simulink model "balanced_modelreduction_rlc"  (R2020b)
settings: Solver=FixedStepAuto  StartTime=0.0  StopTime=3  FixedStep=5e-7  RelTol=1e-3
values from neighbouring files (symbols this model uses):
  n = 20    [Model_1.mat]    (also in Model_11.mat = 100; Model_12.mat = 100; Model_13.mat = 100; Model_14.mat = 100)
undefined symbols (not defined in the file or in its folder): A, Ar, Arg, B, Br, Brg, C, Cr, Crg, K
settings Model: Creator=p282922  LastModifiedBy=S2940884
settings DataIOCC: ReturnWorkspaceOutputs=off
settings DebuggingCC: ArithmeticOperatorsInVariantConditions=warning
settings SFSimCC: SimUseLocalCustomCode=off  CustomCodeUndefinedFunction=UseInterfaceOnly
settings RTWCC: RTWUseLocalCustomCode=off

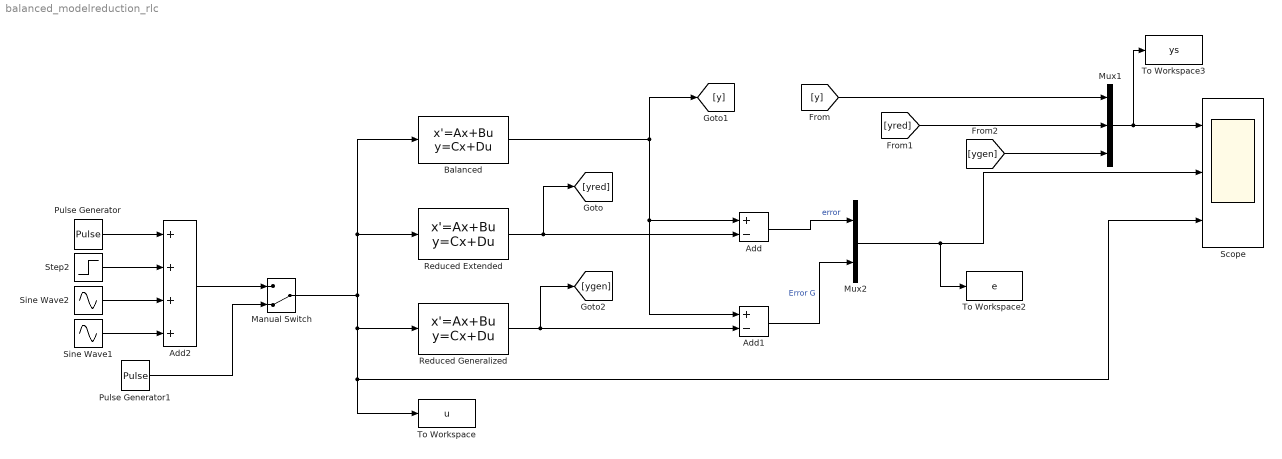
== system balanced_modelreduction_rlc ==
  Add : Sum  Inputs=+-
  Add1 : Sum  Inputs=+-
  Add2 : Sum  Inputs=++++
  Balanced : StateSpace  A=A  B=B  C=C  D=0  InitialCondition=zeros(2*n,1)
  Manual Switch : ManualSwitch  CurrentSetting=0
  Mux1 : Mux  Inputs=3
  Mux2 : Mux  Inputs=2
  Pulse Generator : DiscretePulseGenerator  PulseType=Time based  Amplitude=5  Period=1  PulseWidth=50
  Pulse Generator1 : DiscretePulseGenerator  PulseType=Time based  Amplitude=50  Period=1  PulseWidth=50
  Reduced Extended : StateSpace  A=Ar  B=Br  C=Cr  D=0  InitialCondition=zeros(K,1)
  Reduced Generalized : StateSpace  A=Arg  B=Brg  C=Crg  D=0  InitialCondition=zeros(K,1)
  Scope : Scope  NumInputPorts=3
  Sine Wave1 : Sin  Amplitude=12  Frequency=23  Phase=pi/2  SampleTime=0
  Sine Wave2 : Sin  Amplitude=9  Frequency=17  SampleTime=0
  Step2 : Step  Time=2  After=-30*0  SampleTime=0
  To Workspace : ToWorkspace  VariableName=u  SaveFormat=Structure With Time  SampleTime=-1
  To Workspace2 : ToWorkspace  VariableName=e  SaveFormat=Structure With Time  SampleTime=-1
  To Workspace3 : ToWorkspace  VariableName=ys  SaveFormat=Structure With Time  SampleTime=-1
  wires:
  Balanced/1 -> [y], Add1/1, Add/1
  Reduced Extended/1 -> [yred], Add/2
  Step2/1 -> Add2/2
  [y] -> Mux1/1
  [yred] -> Mux1/2
  Mux1/1 -> To Workspace3/1, Scope/1
  Sine Wave2/1 -> Add2/3
  Pulse Generator/1 -> Add2/1
  Sine Wave1/1 -> Add2/4
  Add2/1 -> Manual Switch/1
  Manual Switch/1 -> Reduced Generalized/1, Scope/3, To Workspace/1, Reduced Extended/1, Balanced/1
  Pulse Generator1/1 -> Manual Switch/2
  Reduced Generalized/1 -> Add1/2, [ygen]
  [ygen] -> Mux1/3
  Add/1 -> Mux2/1  "error"
  Add1/1 -> Mux2/2  "Error G"
  Mux2/1 -> To Workspace2/1, Scope/2
